simulink model "PD_Diagonal"  (R2015a)
settings: Solver=ode4  StartTime=0.0  StopTime=15  RelTol=1e-3
model workspace: external: MAT-File co-effs.mat (data not in the file)
undefined symbols (not defined in the file or in its folder): magnitude
libraries: aerolibutil x104, vrlib x5, dspmathops x4, simulink_extras x2, simulink x1, dspinverses x1
(part 3 of 3)

== system PD_Diagonal/Control Allocation/M3 Distibution/Degress to Volts ==
  X(rad) : Inport
  Y(rad) : Inport  Port=2
  *pi/5 : Constant  Value=pi/5
  0 Point : Constant  Value=2.5
  Sum1 : Sum  Inputs=|++
  Sum4 : Sum  Inputs=++|
  X/180*1 : Product  Inputs=*/
  Y/180*1 : Product  Inputs=*/
  X(V) : Outport
  Y(V) : Outport  Port=2
  wires:
  X(rad)/1 -> X/180*1/1  "X(rad)"
  Y(rad)/1 -> Y/180*1/1  "Y(rad)"
  Sum1/1 -> X(V)/1
  0 Point/1 -> Sum1/2, Sum4/1
  *pi/5/1 -> X/180*1/2, Y/180*1/2
  Sum4/1 -> Y(V)/1
  X/180*1/1 -> Sum1/1
  Y/180*1/1 -> Sum4/2

== system PD_Diagonal/Control Allocation/M3 Distibution/MotorSpeed ==
  F_in : Inport
  Divide : Product  Inputs=*/
  Force Coefficient CT : Constant  Value=0.000243
  Mins : Constant  Value=60
  Product : Product
  w^2 : Sqrt  SaturateOnIntegerOverflow=on
  |F| : Sqrt  SaturateOnIntegerOverflow=on
  |F|^2 : DotProduct  InputSameDT=on  OutDataTypeStr=Inherit: Inherit via internal rule
  RPM : Outport
  wires:
  w^2/1 -> Product/2
  Product/1 -> RPM/1  "RPM"
  Mins/1 -> Product/1
  Divide/1 -> w^2/1
  Force Coefficient CT/1 -> Divide/2
  F_in/1 -> |F|^2/2, |F|^2/1
  |F|^2/1 -> |F|/1
  |F|/1 -> Divide/1

== system PD_Diagonal/Control Allocation/M3 Distibution/Solve M3 XY ==
  Fx : Inport
  Fy : Inport  Port=2
  Fz : Inport  Port=3
  -Fy/T : Gain  Gain=-1
  Constant : Constant  Value=pi
  Dot Product : DotProduct  InputSameDT=on  OutDataTypeStr=Inherit: Inherit via internal rule
  F : Concatenate  NumInputs=3
  Fx/Fz : Product  Inputs=*/
  Fy/T : Product  Inputs=*/
  Sum : Sum  Inputs=|-+
  Switch : Switch  Criteria=u2 > Threshold
  T : Sqrt  Operator=signedSqrt  SaturateOnIntegerOverflow=on
  asin(-Fy/T) : Trigonometry  Operator=asin
  atan(Fx/Fz) : Trigonometry  Operator=atan
  X : Outport
  Y : Outport  Port=2
  wires:
  Fy/1 -> F/2, Fy/T/1
  Fx/1 -> Fx/Fz/1, F/1
  Fz/1 -> F/3, Switch/2, Fx/Fz/2  "Fz"
  F/1 -> Dot Product/2, Dot Product/1
  Dot Product/1 -> T/1
  T/1 -> Fy/T/2  "T"
  asin(-Fy/T)/1 -> Sum/1, Switch/1  "X"
  Switch/1 -> X/1
  Sum/1 -> Switch/3
  Constant/1 -> Sum/2
  atan(Fx/Fz)/1 -> Y/1
  Fy/T/1 -> -Fy/T/1
  -Fy/T/1 -> asin(-Fy/T)/1
  Fx/Fz/1 -> atan(Fx/Fz)/1

== system PD_Diagonal/Control Allocation/M4/M1 DC Motor ==
  note: M1 DC Motor response
  Set Speed(rpm) : Inport
  ->ms : Product  Inputs=*/
  10080 Max : Saturate  UpperLimit=10080  LowerLimit=-10080
  Add : Sum
  Dead Time (ms) : Constant
  Dead Time Block : VariableTransportDelay  MaximumDelay=10
  Miliseconds : Constant  Value=1000
  Starting Speed : Constant  Value=-10080
  Subtract : Sum  Inputs=+-
  Transfer Fcn : TransferFcn  Numerator=1  Denominator=[0.6 1]
  Speed (rpm) : Outport
  wires:
  Dead Time Block/1 -> Transfer Fcn/1
  Miliseconds/1 -> ->ms/2
  Dead Time (ms)/1 -> ->ms/1
  ->ms/1 -> Dead Time Block/2
  Transfer Fcn/1 -> 10080 Max/1
  Set Speed(rpm)/1 -> Subtract/1
  10080 Max/1 -> Add/1
  Add/1 -> Speed (rpm)/1
  Starting Speed/1 -> Subtract/2, Add/2
  Subtract/1 -> Dead Time Block/1

== system PD_Diagonal/Control Allocation/M4/M1 Speed to Thrust ==
  note: RPS to Thrust
  Speed(RPM) : Inport
  ->RPS : Product  Inputs=*/
  Force Coefficient CT : Constant  Value=0.000243
  M1 w^2 : Math  Operator=magnitude^2  SaturateOnIntegerOverflow=on
  Mins : Constant  Value=60
  Product : Product
  Thrust(N) : Outport
  wires:
  M1 w^2/1 -> Product/2
  ->RPS/1 -> M1 w^2/1
  Speed(RPM)/1 -> ->RPS/1
  Force Coefficient CT/1 -> Product/1
  Mins/1 -> ->RPS/2
  Product/1 -> Thrust(N)/1

== system PD_Diagonal/Control Allocation/M4/M1 X Servo  ==
  note: 0V Servo = 0 degree / +90 offset
      | 2.5v Servo = 90 degree/ 0 offset
      | 5v Servo = 180 degree / -90 offset
  note: Servo zero position = 2.5v = 90 degree vertical
  note: 2.5v = 90 degree
  note: 2.5v = 0 offset
  note: M1X Servo Response v->rad
  Input(v) : Inport
  ->ms : Product  Inputs=*/
  ->rad : Constant  Value=pi/5
  Add : Sum  Inputs=+-
  Dead Time (ms) : Constant  Value=3
  Dead Time Block : VariableTransportDelay  MaximumDelay=10
  Default Zero : Constant  Value=pi/2
  Divide : Product  Inputs=*/
  Limits : Constant  OutDataTypeStr=boolean
  Miliseconds : Constant  Value=1000
  Multiply : Product  Inputs=**
  Saturation : Subsystem
  Scope : Scope
      settings: SaveName=ScopeData3
  Starting Position(v) : Constant  Value=2.5
  Subtract : Sum  Inputs=|-+
  Subtract1 : Sum  Inputs=+-|
  Supply (V) : Constant  Value=5
  Transfer Fcn : TransferFcn  Numerator=[pi]  Denominator=[0.11 1]
  Position (rad) : Outport
  wires:
  Miliseconds/1 -> ->ms/2
  Dead Time (ms)/1 -> ->ms/1
  Supply (V)/1 -> Divide/2
  Divide/1 -> Dead Time Block/1
  ->ms/1 -> Dead Time Block/2  "Deadtime 3ms (333hz digital)"
  Dead Time Block/1 -> Transfer Fcn/1
  ->rad/1 -> Multiply/2
  Transfer Fcn/1 -> Saturation/1(Rad)
  Saturation/1(Out1) -> Add/1
  Limits/1 -> Saturation/2(1/0)
  Starting Position(v)/1 -> Multiply/1, Subtract/2
  Subtract/1 -> Divide/1
  Add/1 -> Scope/1, Position (rad)/1
  Multiply/1 -> Subtract1/2
  Input(v)/1 -> Subtract/1
  Subtract1/1 -> Add/2
  Default Zero/1 -> Subtract1/1

== system PD_Diagonal/Control Allocation/M4/M1 Y Servo ==
  note: 0V Servo = 0 degree / +90 offset
      | 2.5v Servo = 90 degree/ 0 offset
      | 5v Servo = 180 degree / -90 offset
  note: Servo zero position = 2.5v = 90 degree vertical
  note: 2.5v = 90 degree
  note: 2.5v = 0 offset
  note: M1Y Servo Response v->rad
  Input(v) : Inport
  ->ms : Product  Inputs=*/
  ->rad : Constant  Value=pi/5
  Add : Sum  Inputs=+-
  Dead Time (ms) : Constant  Value=3
  Dead Time Block : VariableTransportDelay  MaximumDelay=10
  Default Zero : Constant  Value=pi/2
  Divide : Product  Inputs=*/
  Limits : Constant  OutDataTypeStr=boolean
  Miliseconds : Constant  Value=1000
  Multiply : Product  Inputs=**
  Saturation : Subsystem
  Scope : Scope
      settings: SaveName=ScopeData4
  Starting Position(v) : Constant  Value=2.5
  Subtract : Sum  Inputs=|-+
  Subtract1 : Sum  Inputs=+-|
  Supply (V) : Constant  Value=5
  Transfer Fcn : TransferFcn  Numerator=[pi]  Denominator=[0.11 1]
  Position (rad) : Outport
  wires:
  Miliseconds/1 -> ->ms/2
  Dead Time (ms)/1 -> ->ms/1
  Supply (V)/1 -> Divide/2
  Divide/1 -> Dead Time Block/1
  ->ms/1 -> Dead Time Block/2  "Deadtime 3ms (333hz digital)"
  Dead Time Block/1 -> Transfer Fcn/1
  ->rad/1 -> Multiply/2
  Transfer Fcn/1 -> Saturation/1(Rad)
  Saturation/1(Out1) -> Add/1
  Limits/1 -> Saturation/2(1/0)
  Starting Position(v)/1 -> Multiply/1, Subtract/2
  Subtract/1 -> Divide/1
  Add/1 -> Scope/1, Position (rad)/1
  Multiply/1 -> Subtract1/2
  Input(v)/1 -> Subtract/1
  Subtract1/1 -> Add/2
  Default Zero/1 -> Subtract1/1

== system PD_Diagonal/Control Allocation/M4/M1->B Transformation ==
  note: X->Y->Z Transformation Sequence M1->B
  X : Inport
  Y : Inport  Port=2
  "Z " : Inport  Port=3
  Quaternion Multiplication : aerolibutil/Quaternion Multiplication
  Quaternion Multiplication1 : aerolibutil/Quaternion Multiplication
  X Quaternion : Subsystem
  Y Quaternion : Subsystem
  Z Quaternion : Subsystem
  Q_m1 : Outport
  wires:
  X/1 -> X Quaternion/1(y(X Rad))
  "Z "/1 -> Z Quaternion/1(Z Rad)
  Y/1 -> Y Quaternion/1(h(Y Rad))
  Y Quaternion/1(Q_y) -> Quaternion Multiplication/2  "Qy"
  X Quaternion/1(Q_x) -> Quaternion Multiplication/1  "Qx"
  Quaternion Multiplication/1 -> Quaternion Multiplication1/1  "Qx*Qy"
  Z Quaternion/1(Q_z) -> Quaternion Multiplication1/2  "Qz"
  Quaternion Multiplication1/1 -> Q_m1/1  "Qx*Qy*Qz"

== system PD_Diagonal/Control Allocation/M4 Distibution/Degress to Volts ==
  X(rad) : Inport
  Y(rad) : Inport  Port=2
  *pi/5 : Constant  Value=pi/5
  0 Point : Constant  Value=2.5
  Sum1 : Sum  Inputs=|++
  Sum4 : Sum  Inputs=++|
  X/180*1 : Product  Inputs=*/
  Y/180*1 : Product  Inputs=*/
  X(V) : Outport
  Y(V) : Outport  Port=2
  wires:
  X(rad)/1 -> X/180*1/1  "X(rad)"
  Y(rad)/1 -> Y/180*1/1  "Y(rad)"
  Sum1/1 -> X(V)/1
  0 Point/1 -> Sum1/2, Sum4/1
  *pi/5/1 -> X/180*1/2, Y/180*1/2
  Sum4/1 -> Y(V)/1
  X/180*1/1 -> Sum1/1
  Y/180*1/1 -> Sum4/2

== system PD_Diagonal/Control Allocation/M4 Distibution/MotorSpeed ==
  F_in : Inport
  Divide : Product  Inputs=*/
  Force Coefficient CT : Constant  Value=0.000243
  Mins : Constant  Value=60
  Product : Product
  w^2 : Sqrt  SaturateOnIntegerOverflow=on
  |F| : Sqrt  SaturateOnIntegerOverflow=on
  |F|^2 : DotProduct  InputSameDT=on  OutDataTypeStr=Inherit: Inherit via internal rule
  RPM : Outport
  wires:
  w^2/1 -> Product/2
  Product/1 -> RPM/1  "RPM"
  Mins/1 -> Product/1
  Divide/1 -> w^2/1
  Force Coefficient CT/1 -> Divide/2
  F_in/1 -> |F|^2/2, |F|^2/1
  |F|^2/1 -> |F|/1
  |F|/1 -> Divide/1

== system PD_Diagonal/Control Allocation/M4 Distibution/Solve M4 XY ==
  Fx : Inport
  Fy : Inport  Port=2
  Fz : Inport  Port=3
  Constant : Constant  Value=pi
  Dot Product : DotProduct  InputSameDT=on  OutDataTypeStr=Inherit: Inherit via internal rule
  F : Concatenate  NumInputs=3
  Fx/T : Product  Inputs=*/
  Fy/Fz : Product  Inputs=*/
  Sum : Sum  Inputs=|-+
  Switch : Switch  Criteria=u2 > Threshold
  T : Sqrt  Operator=signedSqrt  SaturateOnIntegerOverflow=on
  asin(Fx/T) : Trigonometry  Operator=asin
  atan(Fy/Fz) : Trigonometry  Operator=atan
  X : Outport
  Y : Outport  Port=2
  wires:
  Fy/1 -> Fy/Fz/1, F/2
  Fx/1 -> F/1, Fx/T/1
  Fz/1 -> F/3, Switch/2, Fy/Fz/2  "Fz"
  F/1 -> Dot Product/2, Dot Product/1
  Dot Product/1 -> T/1
  T/1 -> Fx/T/2  "T"
  asin(Fx/T)/1 -> Switch/1, Sum/1  "X"
  Switch/1 -> X/1
  Sum/1 -> Switch/3
  Constant/1 -> Sum/2
  atan(Fy/Fz)/1 -> Y/1
  Fx/T/1 -> asin(Fx/T)/1
  Fy/Fz/1 -> atan(Fy/Fz)/1

== system PD_Diagonal/M1/M1 X Servo /Saturation ==
  note: Switches Satuation Limits
  Rad : Inport
  1/0 : Inport  Port=2
  180 Deg Max : Saturate  UpperLimit=pi  LowerLimit=-pi
  Switch : Switch  Criteria=u2 > Threshold
  Out1 : Outport
  wires:
  180 Deg Max/1 -> Switch/3
  Rad/1 -> Switch/1, 180 Deg Max/1
  Switch/1 -> Out1/1
  1/0/1 -> Switch/2

== system PD_Diagonal/M1/M1 Y Servo/Saturation ==
  note: Switches Satuation Limits
  Rad : Inport
  1/0 : Inport  Port=2
  180 Deg Max : Saturate  UpperLimit=pi  LowerLimit=-pi
  Switch : Switch  Criteria=u2 > Threshold
  Out1 : Outport
  wires:
  180 Deg Max/1 -> Switch/3
  Rad/1 -> Switch/1, 180 Deg Max/1
  Switch/1 -> Out1/1
  1/0/1 -> Switch/2

== system PD_Diagonal/M1/M1->B Transformation/X Quaternion ==
  y(X Rad) : Inport
  Const : Constant  Value=2
  Const1 : Constant  Value=0
  Divide : Product  Inputs=*/
  Trigonometric Function : Trigonometry  Operator=cos
  Trigonometric Function1 : Trigonometry
  Vector Concatenate : Concatenate  NumInputs=4
  Q_x : Outport
  wires:
  Vector Concatenate/1 -> Q_x/1
  Const/1 -> Divide/2
  Trigonometric Function1/1 -> Vector Concatenate/2
  Trigonometric Function/1 -> Vector Concatenate/1
  Const1/1 -> Vector Concatenate/4, Vector Concatenate/3
  Divide/1 -> Trigonometric Function1/1, Trigonometric Function/1
  y(X Rad)/1 -> Divide/1

== system PD_Diagonal/M1/M1->B Transformation/Y Quaternion ==
  h(Y Rad) : Inport
  Const : Constant  Value=2
  Divide : Product  Inputs=*/
  Vector Concatenate : Concatenate  NumInputs=4
  Zero Pad : Constant  Value=0
  cos(Y) : Trigonometry  Operator=cos
  sin(Y) : Trigonometry
  Q_y : Outport
  wires:
  Vector Concatenate/1 -> Q_y/1
  Const/1 -> Divide/2
  cos(Y)/1 -> Vector Concatenate/1
  Zero Pad/1 -> Vector Concatenate/2, Vector Concatenate/4
  Divide/1 -> sin(Y)/1, cos(Y)/1
  sin(Y)/1 -> Vector Concatenate/3
  h(Y Rad)/1 -> Divide/1

== system PD_Diagonal/M1/M1->B Transformation/Z Quaternion ==
  Z Rad : Inport
  Const : Constant  Value=2
  Const1 : Constant  Value=0
  Divide : Product  Inputs=*/
  Trigonometric Function : Trigonometry  Operator=cos
  Trigonometric Function1 : Trigonometry
  Vector Concatenate : Concatenate  NumInputs=4
  Q_z : Outport
  wires:
  Vector Concatenate/1 -> Q_z/1
  Const/1 -> Divide/2
  Trigonometric Function/1 -> Vector Concatenate/1
  Const1/1 -> Vector Concatenate/3, Vector Concatenate/2
  Divide/1 -> Trigonometric Function1/1, Trigonometric Function/1
  Trigonometric Function1/1 -> Vector Concatenate/4
  Z Rad/1 -> Divide/1

== system PD_Diagonal/M2/M2 X Servo /Saturation ==
  note: Switches Satuation Limits
  Rad : Inport
  1/0 : Inport  Port=2
  180 Deg Max : Saturate  UpperLimit=pi  LowerLimit=-pi
  Switch : Switch  Criteria=u2 > Threshold
  Out1 : Outport
  wires:
  180 Deg Max/1 -> Switch/3
  Rad/1 -> Switch/1, 180 Deg Max/1
  Switch/1 -> Out1/1
  1/0/1 -> Switch/2

== system PD_Diagonal/M2/M2 Y Servo/Saturation ==
  note: Switches Satuation Limits
  Rad : Inport
  1/0 : Inport  Port=2
  180 Deg Max : Saturate  UpperLimit=pi  LowerLimit=-pi
  Switch : Switch  Criteria=u2 > Threshold
  Out1 : Outport
  wires:
  180 Deg Max/1 -> Switch/3
  Rad/1 -> Switch/1, 180 Deg Max/1
  Switch/1 -> Out1/1
  1/0/1 -> Switch/2

== system PD_Diagonal/M2/M2->B Transformation/X Quaternion ==
  y(X Rad) : Inport
  Const : Constant  Value=2
  Const1 : Constant  Value=0
  Divide : Product  Inputs=*/
  Trigonometric Function : Trigonometry  Operator=cos
  Trigonometric Function1 : Trigonometry
  Vector Concatenate : Concatenate  NumInputs=4
  Q_x : Outport
  wires:
  Vector Concatenate/1 -> Q_x/1
  Const/1 -> Divide/2
  Trigonometric Function1/1 -> Vector Concatenate/2
  Trigonometric Function/1 -> Vector Concatenate/1
  Const1/1 -> Vector Concatenate/4, Vector Concatenate/3
  Divide/1 -> Trigonometric Function1/1, Trigonometric Function/1
  y(X Rad)/1 -> Divide/1

== system PD_Diagonal/M2/M2->B Transformation/Y Quaternion ==
  h(Y Rad) : Inport
  Const : Constant  Value=2
  Divide : Product  Inputs=*/
  Vector Concatenate : Concatenate  NumInputs=4
  Zero Pad : Constant  Value=0
  cos(Y) : Trigonometry  Operator=cos
  sin(Y) : Trigonometry
  Q_y : Outport
  wires:
  Vector Concatenate/1 -> Q_y/1
  Const/1 -> Divide/2
  cos(Y)/1 -> Vector Concatenate/1
  Zero Pad/1 -> Vector Concatenate/2, Vector Concatenate/4
  Divide/1 -> sin(Y)/1, cos(Y)/1
  sin(Y)/1 -> Vector Concatenate/3
  h(Y Rad)/1 -> Divide/1

== system PD_Diagonal/M2/M2->B Transformation/Z Quaternion ==
  Z Rad : Inport
  Const : Constant  Value=2
  Const1 : Constant  Value=0
  Divide : Product  Inputs=*/
  Trigonometric Function : Trigonometry  Operator=cos
  Trigonometric Function1 : Trigonometry
  Vector Concatenate : Concatenate  NumInputs=4
  Q_z : Outport
  wires:
  Vector Concatenate/1 -> Q_z/1
  Const/1 -> Divide/2
  Trigonometric Function/1 -> Vector Concatenate/1
  Const1/1 -> Vector Concatenate/3, Vector Concatenate/2
  Divide/1 -> Trigonometric Function1/1, Trigonometric Function/1
  Trigonometric Function1/1 -> Vector Concatenate/4
  Z Rad/1 -> Divide/1

== system PD_Diagonal/M3/M3 X Servo /Saturation ==
  note: Switches Satuation Limits
  Rad : Inport
  1/0 : Inport  Port=2
  180 Deg Max : Saturate  UpperLimit=pi  LowerLimit=-pi
  Switch : Switch  Criteria=u2 > Threshold
  Out1 : Outport
  wires:
  180 Deg Max/1 -> Switch/3
  Rad/1 -> Switch/1, 180 Deg Max/1
  Switch/1 -> Out1/1
  1/0/1 -> Switch/2

== system PD_Diagonal/M3/M3 Y Servo/Saturation ==
  note: Switches Satuation Limits
  Rad : Inport
  1/0 : Inport  Port=2
  180 Deg Max : Saturate  UpperLimit=pi  LowerLimit=-pi
  Switch : Switch  Criteria=u2 > Threshold
  Out1 : Outport
  wires:
  180 Deg Max/1 -> Switch/3
  Rad/1 -> Switch/1, 180 Deg Max/1
  Switch/1 -> Out1/1
  1/0/1 -> Switch/2

== system PD_Diagonal/M3/M3->B Transformation/X Quaternion ==
  y(X Rad) : Inport
  Const : Constant  Value=2
  Const1 : Constant  Value=0
  Divide : Product  Inputs=*/
  Trigonometric Function : Trigonometry  Operator=cos
  Trigonometric Function1 : Trigonometry
  Vector Concatenate : Concatenate  NumInputs=4
  Q_x : Outport
  wires:
  Vector Concatenate/1 -> Q_x/1
  Const/1 -> Divide/2
  Trigonometric Function1/1 -> Vector Concatenate/2
  Trigonometric Function/1 -> Vector Concatenate/1
  Const1/1 -> Vector Concatenate/4, Vector Concatenate/3
  Divide/1 -> Trigonometric Function1/1, Trigonometric Function/1
  y(X Rad)/1 -> Divide/1

== system PD_Diagonal/M3/M3->B Transformation/Y Quaternion ==
  h(Y Rad) : Inport
  Const : Constant  Value=2
  Divide : Product  Inputs=*/
  Vector Concatenate : Concatenate  NumInputs=4
  Zero Pad : Constant  Value=0
  cos(Y) : Trigonometry  Operator=cos
  sin(Y) : Trigonometry
  Q_y : Outport
  wires:
  Vector Concatenate/1 -> Q_y/1
  Const/1 -> Divide/2
  cos(Y)/1 -> Vector Concatenate/1
  Zero Pad/1 -> Vector Concatenate/2, Vector Concatenate/4
  Divide/1 -> sin(Y)/1, cos(Y)/1
  sin(Y)/1 -> Vector Concatenate/3
  h(Y Rad)/1 -> Divide/1

== system PD_Diagonal/M3/M3->B Transformation/Z Quaternion ==
  Z Rad : Inport
  Const : Constant  Value=2
  Const1 : Constant  Value=0
  Divide : Product  Inputs=*/
  Trigonometric Function : Trigonometry  Operator=cos
  Trigonometric Function1 : Trigonometry
  Vector Concatenate : Concatenate  NumInputs=4
  Q_z : Outport
  wires:
  Vector Concatenate/1 -> Q_z/1
  Const/1 -> Divide/2
  Trigonometric Function/1 -> Vector Concatenate/1
  Const1/1 -> Vector Concatenate/3, Vector Concatenate/2
  Divide/1 -> Trigonometric Function1/1, Trigonometric Function/1
  Trigonometric Function1/1 -> Vector Concatenate/4
  Z Rad/1 -> Divide/1

== system PD_Diagonal/M4/M4 X Servo /Saturation ==
  note: Switches Satuation Limits
  Rad : Inport
  1/0 : Inport  Port=2
  180 Deg Max : Saturate  UpperLimit=pi  LowerLimit=-pi
  Switch : Switch  Criteria=u2 > Threshold
  Out1 : Outport
  wires:
  180 Deg Max/1 -> Switch/3
  Rad/1 -> Switch/1, 180 Deg Max/1
  Switch/1 -> Out1/1
  1/0/1 -> Switch/2

== system PD_Diagonal/M4/M4 Y Servo/Saturation ==
  note: Switches Satuation Limits
  Rad : Inport
  1/0 : Inport  Port=2
  180 Deg Max : Saturate  UpperLimit=pi  LowerLimit=-pi
  Switch : Switch  Criteria=u2 > Threshold
  Out1 : Outport
  wires:
  180 Deg Max/1 -> Switch/3
  Rad/1 -> Switch/1, 180 Deg Max/1
  Switch/1 -> Out1/1
  1/0/1 -> Switch/2

== system PD_Diagonal/M4/M4->B Transformation/X Quaternion ==
  y(X Rad) : Inport
  Const : Constant  Value=2
  Const1 : Constant  Value=0
  Divide : Product  Inputs=*/
  Trigonometric Function : Trigonometry  Operator=cos
  Trigonometric Function1 : Trigonometry
  Vector Concatenate : Concatenate  NumInputs=4
  Q_x : Outport
  wires:
  Vector Concatenate/1 -> Q_x/1
  Const/1 -> Divide/2
  Trigonometric Function1/1 -> Vector Concatenate/2
  Trigonometric Function/1 -> Vector Concatenate/1
  Const1/1 -> Vector Concatenate/4, Vector Concatenate/3
  Divide/1 -> Trigonometric Function1/1, Trigonometric Function/1
  y(X Rad)/1 -> Divide/1

== system PD_Diagonal/M4/M4->B Transformation/Y Quaternion ==
  h(Y Rad) : Inport
  Const : Constant  Value=2
  Divide : Product  Inputs=*/
  Vector Concatenate : Concatenate  NumInputs=4
  Zero Pad : Constant  Value=0
  cos(Y) : Trigonometry  Operator=cos
  sin(Y) : Trigonometry
  Q_y : Outport
  wires:
  Vector Concatenate/1 -> Q_y/1
  Const/1 -> Divide/2
  cos(Y)/1 -> Vector Concatenate/1
  Zero Pad/1 -> Vector Concatenate/2, Vector Concatenate/4
  Divide/1 -> sin(Y)/1, cos(Y)/1
  sin(Y)/1 -> Vector Concatenate/3
  h(Y Rad)/1 -> Divide/1

== system PD_Diagonal/M4/M4->B Transformation/Z Quaternion ==
  Z Rad : Inport
  Const : Constant  Value=2
  Const1 : Constant  Value=0
  Divide : Product  Inputs=*/
  Trigonometric Function : Trigonometry  Operator=cos
  Trigonometric Function1 : Trigonometry
  Vector Concatenate : Concatenate  NumInputs=4
  Q_z : Outport
  wires:
  Vector Concatenate/1 -> Q_z/1
  Const/1 -> Divide/2
  Trigonometric Function/1 -> Vector Concatenate/1
  Const1/1 -> Vector Concatenate/3, Vector Concatenate/2
  Divide/1 -> Trigonometric Function1/1, Trigonometric Function/1
  Trigonometric Function1/1 -> Vector Concatenate/4
  Z Rad/1 -> Divide/1

== system PD_Diagonal/t_M/M1 Torque/M Quaternion ==
  h(Y Rad) : Inport
  Const : Constant  Value=2
  Divide : Product  Inputs=*/
  Vector Concatenate : Concatenate  NumInputs=4
  Zero Pad : Constant  Value=0
  cos(Y) : Trigonometry  Operator=cos
  sin(Y) : Trigonometry
  Q_y : Outport
  wires:
  Vector Concatenate/1 -> Q_y/1
  Const/1 -> Divide/2
  cos(Y)/1 -> Vector Concatenate/1
  Zero Pad/1 -> Vector Concatenate/2, Vector Concatenate/4
  Divide/1 -> sin(Y)/1, cos(Y)/1
  sin(Y)/1 -> Vector Concatenate/3
  h(Y Rad)/1 -> Divide/1

== system PD_Diagonal/t_M/M1 Torque/Ring Quaternion ==
  y(X Rad) : Inport
  Const : Constant  Value=2
  Const1 : Constant  Value=0
  Divide : Product  Inputs=*/
  Trigonometric Function : Trigonometry  Operator=cos
  Trigonometric Function1 : Trigonometry
  Vector Concatenate : Concatenate  NumInputs=4
  Q_R : Outport
  wires:
  Vector Concatenate/1 -> Q_R/1
  Const/1 -> Divide/2
  Trigonometric Function1/1 -> Vector Concatenate/2
  Trigonometric Function/1 -> Vector Concatenate/1
  Const1/1 -> Vector Concatenate/4, Vector Concatenate/3
  Divide/1 -> Trigonometric Function1/1, Trigonometric Function/1
  y(X Rad)/1 -> Divide/1

== system PD_Diagonal/t_M/M1 Torque/Z Quaternion ==
  Z Rad : Inport
  Const : Constant  Value=2
  Const1 : Constant  Value=0
  Divide : Product  Inputs=*/
  Trigonometric Function : Trigonometry  Operator=cos
  Trigonometric Function1 : Trigonometry
  Vector Concatenate : Concatenate  NumInputs=4
  Q_z : Outport
  wires:
  Vector Concatenate/1 -> Q_z/1
  Const/1 -> Divide/2
  Trigonometric Function/1 -> Vector Concatenate/1
  Const1/1 -> Vector Concatenate/3, Vector Concatenate/2
  Divide/1 -> Trigonometric Function1/1, Trigonometric Function/1
  Trigonometric Function1/1 -> Vector Concatenate/4
  Z Rad/1 -> Divide/1

== system PD_Diagonal/t_M/M2 Torque/M Quaternion ==
  h(Y Rad) : Inport
  Const : Constant  Value=2
  Divide : Product  Inputs=*/
  Vector Concatenate : Concatenate  NumInputs=4
  Zero Pad : Constant  Value=0
  cos(Y) : Trigonometry  Operator=cos
  sin(Y) : Trigonometry
  Q_y : Outport
  wires:
  Vector Concatenate/1 -> Q_y/1
  Const/1 -> Divide/2
  cos(Y)/1 -> Vector Concatenate/1
  Zero Pad/1 -> Vector Concatenate/2, Vector Concatenate/4
  Divide/1 -> sin(Y)/1, cos(Y)/1
  sin(Y)/1 -> Vector Concatenate/3
  h(Y Rad)/1 -> Divide/1

== system PD_Diagonal/t_M/M2 Torque/Ring Quaternion ==
  y(X Rad) : Inport
  Const : Constant  Value=2
  Const1 : Constant  Value=0
  Divide : Product  Inputs=*/
  Trigonometric Function : Trigonometry  Operator=cos
  Trigonometric Function1 : Trigonometry
  Vector Concatenate : Concatenate  NumInputs=4
  Q_R : Outport
  wires:
  Vector Concatenate/1 -> Q_R/1
  Const/1 -> Divide/2
  Trigonometric Function1/1 -> Vector Concatenate/2
  Trigonometric Function/1 -> Vector Concatenate/1
  Const1/1 -> Vector Concatenate/4, Vector Concatenate/3
  Divide/1 -> Trigonometric Function1/1, Trigonometric Function/1
  y(X Rad)/1 -> Divide/1

== system PD_Diagonal/t_M/M2 Torque/Z Quaternion ==
  Z Rad : Inport
  Const : Constant  Value=2
  Const1 : Constant  Value=0
  Divide : Product  Inputs=*/
  Trigonometric Function : Trigonometry  Operator=cos
  Trigonometric Function1 : Trigonometry
  Vector Concatenate : Concatenate  NumInputs=4
  Q_z : Outport
  wires:
  Vector Concatenate/1 -> Q_z/1
  Const/1 -> Divide/2
  Trigonometric Function/1 -> Vector Concatenate/1
  Const1/1 -> Vector Concatenate/3, Vector Concatenate/2
  Divide/1 -> Trigonometric Function1/1, Trigonometric Function/1
  Trigonometric Function1/1 -> Vector Concatenate/4
  Z Rad/1 -> Divide/1

== system PD_Diagonal/t_M/M3 Torque/M Quaternion ==
  h(Y Rad) : Inport
  Const : Constant  Value=2
  Divide : Product  Inputs=*/
  Vector Concatenate : Concatenate  NumInputs=4
  Zero Pad : Constant  Value=0
  cos(Y) : Trigonometry  Operator=cos
  sin(Y) : Trigonometry
  Q_y : Outport
  wires:
  Vector Concatenate/1 -> Q_y/1
  Const/1 -> Divide/2
  cos(Y)/1 -> Vector Concatenate/1
  Zero Pad/1 -> Vector Concatenate/2, Vector Concatenate/4
  Divide/1 -> sin(Y)/1, cos(Y)/1
  sin(Y)/1 -> Vector Concatenate/3
  h(Y Rad)/1 -> Divide/1

== system PD_Diagonal/t_M/M3 Torque/Ring Quaternion ==
  y(X Rad) : Inport
  Const : Constant  Value=2
  Const1 : Constant  Value=0
  Divide : Product  Inputs=*/
  Trigonometric Function : Trigonometry  Operator=cos
  Trigonometric Function1 : Trigonometry
  Vector Concatenate : Concatenate  NumInputs=4
  Q_R : Outport
  wires:
  Vector Concatenate/1 -> Q_R/1
  Const/1 -> Divide/2
  Trigonometric Function1/1 -> Vector Concatenate/2
  Trigonometric Function/1 -> Vector Concatenate/1
  Const1/1 -> Vector Concatenate/4, Vector Concatenate/3
  Divide/1 -> Trigonometric Function1/1, Trigonometric Function/1
  y(X Rad)/1 -> Divide/1

== system PD_Diagonal/t_M/M3 Torque/Z Quaternion ==
  Z Rad : Inport
  Const : Constant  Value=2
  Const1 : Constant  Value=0
  Divide : Product  Inputs=*/
  Trigonometric Function : Trigonometry  Operator=cos
  Trigonometric Function1 : Trigonometry
  Vector Concatenate : Concatenate  NumInputs=4
  Q_z : Outport
  wires:
  Vector Concatenate/1 -> Q_z/1
  Const/1 -> Divide/2
  Trigonometric Function/1 -> Vector Concatenate/1
  Const1/1 -> Vector Concatenate/3, Vector Concatenate/2
  Divide/1 -> Trigonometric Function1/1, Trigonometric Function/1
  Trigonometric Function1/1 -> Vector Concatenate/4
  Z Rad/1 -> Divide/1

== system PD_Diagonal/t_M/M4 Torque/M Quaternion ==
  h(Y Rad) : Inport
  Const : Constant  Value=2
  Divide : Product  Inputs=*/
  Vector Concatenate : Concatenate  NumInputs=4
  Zero Pad : Constant  Value=0
  cos(Y) : Trigonometry  Operator=cos
  sin(Y) : Trigonometry
  Q_y : Outport
  wires:
  Vector Concatenate/1 -> Q_y/1
  Const/1 -> Divide/2
  cos(Y)/1 -> Vector Concatenate/1
  Zero Pad/1 -> Vector Concatenate/2, Vector Concatenate/4
  Divide/1 -> sin(Y)/1, cos(Y)/1
  sin(Y)/1 -> Vector Concatenate/3
  h(Y Rad)/1 -> Divide/1

== system PD_Diagonal/t_M/M4 Torque/Ring Quaternion ==
  y(X Rad) : Inport
  Const : Constant  Value=2
  Const1 : Constant  Value=0
  Divide : Product  Inputs=*/
  Trigonometric Function : Trigonometry  Operator=cos
  Trigonometric Function1 : Trigonometry
  Vector Concatenate : Concatenate  NumInputs=4
  Q_R : Outport
  wires:
  Vector Concatenate/1 -> Q_R/1
  Const/1 -> Divide/2
  Trigonometric Function1/1 -> Vector Concatenate/2
  Trigonometric Function/1 -> Vector Concatenate/1
  Const1/1 -> Vector Concatenate/4, Vector Concatenate/3
  Divide/1 -> Trigonometric Function1/1, Trigonometric Function/1
  y(X Rad)/1 -> Divide/1

== system PD_Diagonal/t_M/M4 Torque/Z Quaternion ==
  Z Rad : Inport
  Const : Constant  Value=2
  Const1 : Constant  Value=0
  Divide : Product  Inputs=*/
  Trigonometric Function : Trigonometry  Operator=cos
  Trigonometric Function1 : Trigonometry
  Vector Concatenate : Concatenate  NumInputs=4
  Q_z : Outport
  wires:
  Vector Concatenate/1 -> Q_z/1
  Const/1 -> Divide/2
  Trigonometric Function/1 -> Vector Concatenate/1
  Const1/1 -> Vector Concatenate/3, Vector Concatenate/2
  Divide/1 -> Trigonometric Function1/1, Trigonometric Function/1
  Trigonometric Function1/1 -> Vector Concatenate/4
  Z Rad/1 -> Divide/1

== system PD_Diagonal/Control Allocation/M1/M1 X Servo /Saturation ==
  note: Switches Satuation Limits
  Rad : Inport
  1/0 : Inport  Port=2
  180 Deg Max : Saturate  UpperLimit=pi  LowerLimit=-pi
  Display : Display
  Switch : Switch  Criteria=u2 > Threshold
  Out1 : Outport
  wires:
  180 Deg Max/1 -> Switch/3
  Rad/1 -> Switch/1, 180 Deg Max/1
  Switch/1 -> Out1/1
  1/0/1 -> Switch/2

== system PD_Diagonal/Control Allocation/M1/M1 Y Servo/Saturation ==
  note: Switches Satuation Limits
  Rad : Inport
  1/0 : Inport  Port=2
  180 Deg Max : Saturate  UpperLimit=pi  LowerLimit=-pi
  Switch : Switch  Criteria=u2 > Threshold
  Out1 : Outport
  wires:
  180 Deg Max/1 -> Switch/3
  Rad/1 -> Switch/1, 180 Deg Max/1
  Switch/1 -> Out1/1
  1/0/1 -> Switch/2

== system PD_Diagonal/Control Allocation/M1/M1->B Transformation/X Quaternion ==
  y(X Rad) : Inport
  Const : Constant  Value=2
  Const1 : Constant  Value=0
  Divide : Product  Inputs=*/
  Trigonometric Function : Trigonometry  Operator=cos
  Trigonometric Function1 : Trigonometry
  Vector Concatenate : Concatenate  NumInputs=4
  Q_x : Outport
  wires:
  Vector Concatenate/1 -> Q_x/1
  Const/1 -> Divide/2
  Trigonometric Function1/1 -> Vector Concatenate/2
  Trigonometric Function/1 -> Vector Concatenate/1
  Const1/1 -> Vector Concatenate/4, Vector Concatenate/3
  Divide/1 -> Trigonometric Function1/1, Trigonometric Function/1
  y(X Rad)/1 -> Divide/1

== system PD_Diagonal/Control Allocation/M1/M1->B Transformation/Y Quaternion ==
  h(Y Rad) : Inport
  Const : Constant  Value=2
  Divide : Product  Inputs=*/
  Vector Concatenate : Concatenate  NumInputs=4
  Zero Pad : Constant  Value=0
  cos(Y) : Trigonometry  Operator=cos
  sin(Y) : Trigonometry
  Q_y : Outport
  wires:
  Vector Concatenate/1 -> Q_y/1
  Const/1 -> Divide/2
  cos(Y)/1 -> Vector Concatenate/1
  Zero Pad/1 -> Vector Concatenate/2, Vector Concatenate/4
  Divide/1 -> sin(Y)/1, cos(Y)/1
  sin(Y)/1 -> Vector Concatenate/3
  h(Y Rad)/1 -> Divide/1

== system PD_Diagonal/Control Allocation/M1/M1->B Transformation/Z Quaternion ==
  Z Rad : Inport
  Const : Constant  Value=2
  Const1 : Constant  Value=0
  Divide : Product  Inputs=*/
  Trigonometric Function : Trigonometry  Operator=cos
  Trigonometric Function1 : Trigonometry
  Vector Concatenate : Concatenate  NumInputs=4
  Q_z : Outport
  wires:
  Vector Concatenate/1 -> Q_z/1
  Const/1 -> Divide/2
  Trigonometric Function/1 -> Vector Concatenate/1
  Const1/1 -> Vector Concatenate/3, Vector Concatenate/2
  Divide/1 -> Trigonometric Function1/1, Trigonometric Function/1
  Trigonometric Function1/1 -> Vector Concatenate/4
  Z Rad/1 -> Divide/1

== system PD_Diagonal/Control Allocation/M2/M1 X Servo /Saturation ==
  note: Switches Satuation Limits
  Rad : Inport
  1/0 : Inport  Port=2
  180 Deg Max : Saturate  UpperLimit=pi  LowerLimit=-pi
  Display : Display
  Switch : Switch  Criteria=u2 > Threshold
  Out1 : Outport
  wires:
  180 Deg Max/1 -> Switch/3
  Rad/1 -> Switch/1, 180 Deg Max/1
  Switch/1 -> Out1/1
  1/0/1 -> Switch/2

== system PD_Diagonal/Control Allocation/M2/M1 Y Servo/Saturation ==
  note: Switches Satuation Limits
  Rad : Inport
  1/0 : Inport  Port=2
  180 Deg Max : Saturate  UpperLimit=pi  LowerLimit=-pi
  Switch : Switch  Criteria=u2 > Threshold
  Out1 : Outport
  wires:
  180 Deg Max/1 -> Switch/3
  Rad/1 -> Switch/1, 180 Deg Max/1
  Switch/1 -> Out1/1
  1/0/1 -> Switch/2

== system PD_Diagonal/Control Allocation/M2/M1->B Transformation/X Quaternion ==
  y(X Rad) : Inport
  Const : Constant  Value=2
  Const1 : Constant  Value=0
  Divide : Product  Inputs=*/
  Trigonometric Function : Trigonometry  Operator=cos
  Trigonometric Function1 : Trigonometry
  Vector Concatenate : Concatenate  NumInputs=4
  Q_x : Outport
  wires:
  Vector Concatenate/1 -> Q_x/1
  Const/1 -> Divide/2
  Trigonometric Function1/1 -> Vector Concatenate/2
  Trigonometric Function/1 -> Vector Concatenate/1
  Const1/1 -> Vector Concatenate/4, Vector Concatenate/3
  Divide/1 -> Trigonometric Function1/1, Trigonometric Function/1
  y(X Rad)/1 -> Divide/1

== system PD_Diagonal/Control Allocation/M2/M1->B Transformation/Y Quaternion ==
  h(Y Rad) : Inport
  Const : Constant  Value=2
  Divide : Product  Inputs=*/
  Vector Concatenate : Concatenate  NumInputs=4
  Zero Pad : Constant  Value=0
  cos(Y) : Trigonometry  Operator=cos
  sin(Y) : Trigonometry
  Q_y : Outport
  wires:
  Vector Concatenate/1 -> Q_y/1
  Const/1 -> Divide/2
  cos(Y)/1 -> Vector Concatenate/1
  Zero Pad/1 -> Vector Concatenate/2, Vector Concatenate/4
  Divide/1 -> sin(Y)/1, cos(Y)/1
  sin(Y)/1 -> Vector Concatenate/3
  h(Y Rad)/1 -> Divide/1

== system PD_Diagonal/Control Allocation/M2/M1->B Transformation/Z Quaternion ==
  Z Rad : Inport
  Const : Constant  Value=2
  Const1 : Constant  Value=0
  Divide : Product  Inputs=*/
  Trigonometric Function : Trigonometry  Operator=cos
  Trigonometric Function1 : Trigonometry
  Vector Concatenate : Concatenate  NumInputs=4
  Q_z : Outport
  wires:
  Vector Concatenate/1 -> Q_z/1
  Const/1 -> Divide/2
  Trigonometric Function/1 -> Vector Concatenate/1
  Const1/1 -> Vector Concatenate/3, Vector Concatenate/2
  Divide/1 -> Trigonometric Function1/1, Trigonometric Function/1
  Trigonometric Function1/1 -> Vector Concatenate/4
  Z Rad/1 -> Divide/1

== system PD_Diagonal/Control Allocation/M3/M1 X Servo /Saturation ==
  note: Switches Satuation Limits
  Rad : Inport
  1/0 : Inport  Port=2
  180 Deg Max : Saturate  UpperLimit=pi  LowerLimit=-pi
  Display : Display
  Switch : Switch  Criteria=u2 > Threshold
  Out1 : Outport
  wires:
  180 Deg Max/1 -> Switch/3
  Rad/1 -> Switch/1, 180 Deg Max/1
  Switch/1 -> Out1/1
  1/0/1 -> Switch/2

== system PD_Diagonal/Control Allocation/M3/M1 Y Servo/Saturation ==
  note: Switches Satuation Limits
  Rad : Inport
  1/0 : Inport  Port=2
  180 Deg Max : Saturate  UpperLimit=pi  LowerLimit=-pi
  Switch : Switch  Criteria=u2 > Threshold
  Out1 : Outport
  wires:
  180 Deg Max/1 -> Switch/3
  Rad/1 -> Switch/1, 180 Deg Max/1
  Switch/1 -> Out1/1
  1/0/1 -> Switch/2

== system PD_Diagonal/Control Allocation/M3/M1->B Transformation/X Quaternion ==
  y(X Rad) : Inport
  Const : Constant  Value=2
  Const1 : Constant  Value=0
  Divide : Product  Inputs=*/
  Trigonometric Function : Trigonometry  Operator=cos
  Trigonometric Function1 : Trigonometry
  Vector Concatenate : Concatenate  NumInputs=4
  Q_x : Outport
  wires:
  Vector Concatenate/1 -> Q_x/1
  Const/1 -> Divide/2
  Trigonometric Function1/1 -> Vector Concatenate/2
  Trigonometric Function/1 -> Vector Concatenate/1
  Const1/1 -> Vector Concatenate/4, Vector Concatenate/3
  Divide/1 -> Trigonometric Function1/1, Trigonometric Function/1
  y(X Rad)/1 -> Divide/1

== system PD_Diagonal/Control Allocation/M3/M1->B Transformation/Y Quaternion ==
  h(Y Rad) : Inport
  Const : Constant  Value=2
  Divide : Product  Inputs=*/
  Vector Concatenate : Concatenate  NumInputs=4
  Zero Pad : Constant  Value=0
  cos(Y) : Trigonometry  Operator=cos
  sin(Y) : Trigonometry
  Q_y : Outport
  wires:
  Vector Concatenate/1 -> Q_y/1
  Const/1 -> Divide/2
  cos(Y)/1 -> Vector Concatenate/1
  Zero Pad/1 -> Vector Concatenate/2, Vector Concatenate/4
  Divide/1 -> sin(Y)/1, cos(Y)/1
  sin(Y)/1 -> Vector Concatenate/3
  h(Y Rad)/1 -> Divide/1

== system PD_Diagonal/Control Allocation/M3/M1->B Transformation/Z Quaternion ==
  Z Rad : Inport
  Const : Constant  Value=2
  Const1 : Constant  Value=0
  Divide : Product  Inputs=*/
  Trigonometric Function : Trigonometry  Operator=cos
  Trigonometric Function1 : Trigonometry
  Vector Concatenate : Concatenate  NumInputs=4
  Q_z : Outport
  wires:
  Vector Concatenate/1 -> Q_z/1
  Const/1 -> Divide/2
  Trigonometric Function/1 -> Vector Concatenate/1
  Const1/1 -> Vector Concatenate/3, Vector Concatenate/2
  Divide/1 -> Trigonometric Function1/1, Trigonometric Function/1
  Trigonometric Function1/1 -> Vector Concatenate/4
  Z Rad/1 -> Divide/1

== system PD_Diagonal/Control Allocation/M4/M1 X Servo /Saturation ==
  note: Switches Satuation Limits
  Rad : Inport
  1/0 : Inport  Port=2
  180 Deg Max : Saturate  UpperLimit=pi  LowerLimit=-pi
  Display : Display
  Switch : Switch  Criteria=u2 > Threshold
  Out1 : Outport
  wires:
  180 Deg Max/1 -> Switch/3
  Rad/1 -> Switch/1, 180 Deg Max/1
  Switch/1 -> Out1/1
  1/0/1 -> Switch/2

== system PD_Diagonal/Control Allocation/M4/M1 Y Servo/Saturation ==
  note: Switches Satuation Limits
  Rad : Inport
  1/0 : Inport  Port=2
  180 Deg Max : Saturate  UpperLimit=pi  LowerLimit=-pi
  Switch : Switch  Criteria=u2 > Threshold
  Out1 : Outport
  wires:
  180 Deg Max/1 -> Switch/3
  Rad/1 -> Switch/1, 180 Deg Max/1
  Switch/1 -> Out1/1
  1/0/1 -> Switch/2

== system PD_Diagonal/Control Allocation/M4/M1->B Transformation/X Quaternion ==
  y(X Rad) : Inport
  Const : Constant  Value=2
  Const1 : Constant  Value=0
  Divide : Product  Inputs=*/
  Trigonometric Function : Trigonometry  Operator=cos
  Trigonometric Function1 : Trigonometry
  Vector Concatenate : Concatenate  NumInputs=4
  Q_x : Outport
  wires:
  Vector Concatenate/1 -> Q_x/1
  Const/1 -> Divide/2
  Trigonometric Function1/1 -> Vector Concatenate/2
  Trigonometric Function/1 -> Vector Concatenate/1
  Const1/1 -> Vector Concatenate/4, Vector Concatenate/3
  Divide/1 -> Trigonometric Function1/1, Trigonometric Function/1
  y(X Rad)/1 -> Divide/1

== system PD_Diagonal/Control Allocation/M4/M1->B Transformation/Y Quaternion ==
  h(Y Rad) : Inport
  Const : Constant  Value=2
  Divide : Product  Inputs=*/
  Vector Concatenate : Concatenate  NumInputs=4
  Zero Pad : Constant  Value=0
  cos(Y) : Trigonometry  Operator=cos
  sin(Y) : Trigonometry
  Q_y : Outport
  wires:
  Vector Concatenate/1 -> Q_y/1
  Const/1 -> Divide/2
  cos(Y)/1 -> Vector Concatenate/1
  Zero Pad/1 -> Vector Concatenate/2, Vector Concatenate/4
  Divide/1 -> sin(Y)/1, cos(Y)/1
  sin(Y)/1 -> Vector Concatenate/3
  h(Y Rad)/1 -> Divide/1

== system PD_Diagonal/Control Allocation/M4/M1->B Transformation/Z Quaternion ==
  Z Rad : Inport
  Const : Constant  Value=2
  Const1 : Constant  Value=0
  Divide : Product  Inputs=*/
  Trigonometric Function : Trigonometry  Operator=cos
  Trigonometric Function1 : Trigonometry
  Vector Concatenate : Concatenate  NumInputs=4
  Q_z : Outport
  wires:
  Vector Concatenate/1 -> Q_z/1
  Const/1 -> Divide/2
  Trigonometric Function/1 -> Vector Concatenate/1
  Const1/1 -> Vector Concatenate/3, Vector Concatenate/2
  Divide/1 -> Trigonometric Function1/1, Trigonometric Function/1
  Trigonometric Function1/1 -> Vector Concatenate/4
  Z Rad/1 -> Divide/1

== matlab function PD_Diagonal/Plot/Plot Function ==
  data: q input; e1 input; t input; l input; pr input; qmtr1 input; qmtr2 input; qmtr3 input; qmtr4 input
function plot(q,e1,t,l,pr,qmtr1,qmtr2,qmtr3,qmtr4)
%Input t
%CG Cartesian Co-ordinates
X = e1(1); %X Position
Y = e1(2); %Y Position
Z = e1(3); %Z Position
%Calculate Motor Positions relative to 0;0;0
%l may be variable
XYmtr1 = (l/sqrt(2))*([1 1 0]);
XYmtr2 = (l/sqrt(2))*([-1 1 0]);
XYmtr3 = (l/sqrt(2))*([-1 -1 0]);
XYmtr4 = (l/sqrt(2))*([1 -1 0]);
%%Calculate Body Attidue (Normal Vector)
Q = quatnormalize(q.'); %Body Quaternion, read from d/dt(Q)
Q_conj = quatconj(Q);   %Quaternion conjugate
N_b = [0 0 1];      %normal vector in Body frame
L_b = [0 N_b(1) N_b(2) N_b(3)]; %Build normal quaternion
L1 = quatmultiply(Q_conj,L_b);
L2 = quatmultiply(L1,Q);    %Normal rotated by Body Quaternion
N_w = [L2(2) L2(3) L2(4)];  %Normal vector in inertial frame
%%Calculate Motor 1 Attitudes
Q_XYmtr1 = [0 XYmtr1(1) XYmtr1(2) XYmtr1(3)]; %XYZ position of motor 1 from CG
L1 = quatmultiply(Q_conj,Q_XYmtr1);
L2 = quatmultiply(L1,Q);    %Rotate rotor arm by body quaternion
mtr1_w = e1.' + [L2(2) L2(3) L2(4)]; %Calculate new XYZ position using attitude quaternion
L_1 = [0 0 0 1];       %k considered to be normal for motor 1 (Force acting just in the Z-direction)
Q_mtr1 = [qmtr1(1) qmtr1(2) qmtr1(3) qmtr1(4)]; %Calculate motor 1 attitude from motor 1 quaternion
Q_mtr1_conj = quatconj(Q_mtr1);
L1 = quatmultiply(Q_mtr1_conj,L_1);
L2 = quatmultiply(L1,Q_mtr1);
L3 = quatmultiply(Q_conj,L2);
L4 = quatmultiply(L3,Q);
mtr1_N = [L4(2) L4(3) L4(4)]; %Motor 1 Normal Vector
%%Calculate Motor 3 Attitudes
Q_XYmtr3 = [0 XYmtr3(1) XYmtr3(2) XYmtr3(3)];
L1 = quatmultiply(Q_conj,Q_XYmtr3);
L2 = quatmultiply(L1,Q);
mtr3_w = e1.' + [L2(2) L2(3) L2(4)];
L_3 = [0 0 0 1];
Q_mtr3 = [qmtr3(1) qmtr3(2) qmtr3(3) qmtr3(4)]; %Calculate motor 3 attitude from motor 3 quaternion
Q_mtr3_conj = quatconj(Q_mtr3);
L1 = quatmultiply(Q_mtr3_conj,L_3);
L2 = quatmultiply(L1,Q_mtr3);
L3 = quatmultiply(Q_conj,L2);
L4 = quatmultiply(L3,Q);
mtr3_N = [L4(2) L4(3) L4(4)]; %Motor 3 Normal Vector
%%Calculate Motor 2 Attitudes
Q_XYmtr2 = [0 XYmtr2(1) XYmtr2(2) XYmtr2(3)];
L1 = quatmultiply(Q_conj,Q_XYmtr2);
L2 = quatmultiply(L1,Q);
mtr2_w = e1.' + [L2(2) L2(3) L2(4)];
L_2 = [0 0 0 1];
Q_mtr2 = [qmtr2(1) qmtr2(2) qmtr2(3) qmtr2(4)]; %Calculate motor 2 attitude from motor 2 quaternion
Q_mtr2_conj = quatconj(Q_mtr2);
L1 = quatmultiply(Q_mtr2_conj,L_2);
L2 = quatmultiply(L1,Q_mtr2);
L3 = quatmultiply(Q_conj,L2);
L4 = quatmultiply(L3,Q);
mtr2_N = [L4(2) L4(3) L4(4)]; %Motor 2 Normal Vector
%%Calculate Motor 4 Attitudes
Q_XYmtr4 = [0 XYmtr4(1) XYmtr4(2) XYmtr4(3)];
L1 = quatmultiply(Q_conj,Q_XYmtr4);
L2 = quatmultiply(L1,Q);
mtr4_w = e1.' + [L2(2) L2(3) L2(4)];
L_4 = [0 0 0 1];
Q_mtr4 = [qmtr4(1) qmtr4(2) qmtr4(3) qmtr4(4)]; %Calculate motor 2 attitude from motor 2 quaternion
Q_mtr4_conj = quatconj(Q_mtr4);
L1 = quatmultiply(Q_mtr4_conj,L_4);
L2 = quatmultiply(L1,Q_mtr4);
L3 = quatmultiply(Q_conj,L2);
L4 = quatmultiply(L3,Q);
mtr4_N = [L4(2) L4(3) L4(4)]; %Motor 2 Normal Vector
%%Open Figure if first time instance
if(t==0);
    fig = figure();
    hold on;
    grid on;
end
%%Clear and Construct Figure
hold off;
clf();
xlim([-1 5]);
ylim([-1 5]);
zlim([0 5]);
view([2,2,4]);
grid on;
hold on;
%%Display Time
%disp(t);
%%Plot Quad Function
plotCircle3D([X Y 0],[0 0 1],(l),'black');
N = e1.' + 1*N_w;
plot3(([e1(1) N(1)]),([e1(2) N(2)]),([e1(3) N(3)]),'LineWidth',1,'Color','green');
plot3(([mtr1_w(1) mtr3_w(1)]),([mtr1_w(2) mtr3_w(2)]),([mtr1_w(3) mtr3_w(3)]),'LineWidth',1,'Color','Blue');
plot3(([mtr2_w(1) mtr4_w(1)]),([mtr2_w(2) mtr4_w(2)]),([mtr2_w(3) mtr4_w(3)]),'LineWidth',1,'Color','Blue');
plotCircle3D(mtr1_w,mtr1_N,pr,'red');
plotCircle3D(mtr2_w,mtr2_N,pr,'red');
plotCircle3D(mtr3_w,mtr3_N,pr,'red');
plotCircle3D(mtr4_w,mtr4_N,pr,'red');
plotCircle3D([X Y Z],N_w,(l+pr),'green');
%%
end
